simulink model "T_DARM_Functional_Architecture"  (R2021a)
settings: Solver=VariableStepAuto  StartTime=0.0  StopTime=10.0  RelTol=1e-3
settings Model: Creator=Daniel Adejumo  LastModifiedBy=Daniel Adejumo

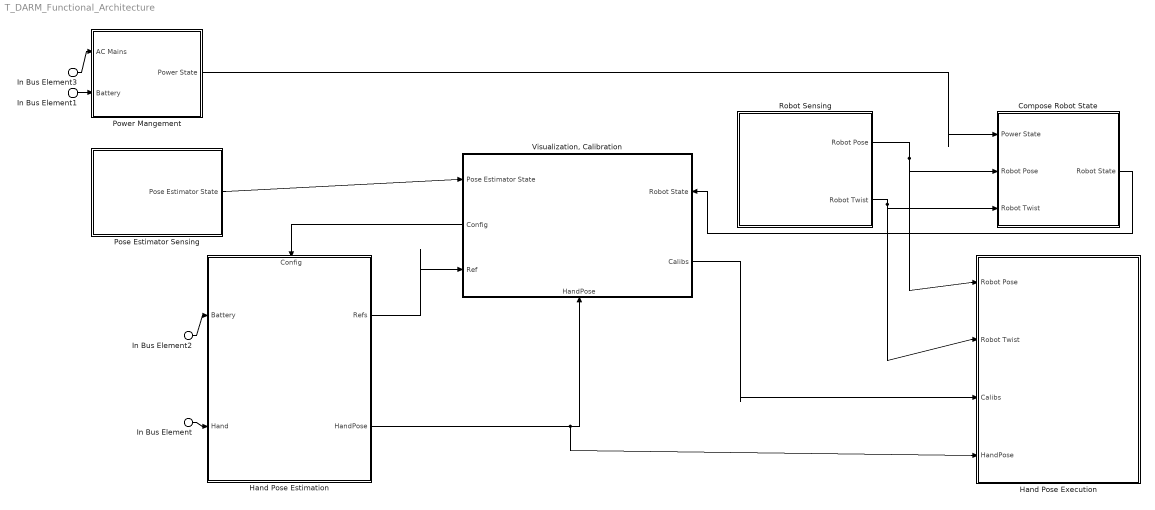
== system T_DARM_Functional_Architecture ==
  In Bus Element3 : Inport  PortName=AC Mains
  In Bus Element2 : Inport  Port=2  PortName=Battery
  In Bus Element1 : Inport  Port=2  PortName=Battery
  In Bus Element : Inport  Port=3  PortName=Hand
  Compose Robot State : Subsystem
      settings: PortSchema="{\"entries\":[{\"content\":{\"headerSize\":26,\"margin\":15,\"minimumSpacing\":25,\"sides\":[{\"content\":{\"connectorIds\":[\"In1\",\"In2\",\"In3\"]},\"type\":\"ConnectorPlacement.EquallySpacedRectSide\",\"uuid\":\"05d6e9f9-85ca-4a6e-a9b5-67e652ad81e0\"},{\"content\":{\"connectorIds\":[\"Out1\"],\"side\":\"RIGHT\"},\"type\":\"ConnectorPlacement.EquallySpacedRectSide\",\"uuid\":\"e4d931d8-63a7-4c55-9fa4-e3388543b788\"},{\"content\":{\"connectorIds\":[],\"side\":\"TOP\"},\"type\":\"ConnectorPlacement.EquallySpacedRectSide\",\"uuid\":\"0b7a612c-5d49-405f-8f52-91f0f155fa8d\"}]},\"type\":\"ConnectorPlacement.EquallySpacedConnector\",\"uuid\":\"d040a7c1-518a-4586-9505-55d0b93cd332\"}],\"packageUris\":[\"http://schema.mathworks.com/mf0/Connector/R2020b\"],\"version\":\"1.0\"}"
  Hand Pose Estimation : Subsystem
      settings: PortSchema="{\"entries\":[{\"content\":{\"headerSize\":26,\"margin\":15,\"minimumSpacing\":25,\"sides\":[{\"content\":{\"connectorIds\":[\"In2\",\"In3\"]},\"type\":\"ConnectorPlacement.EquallySpacedRectSide\",\"uuid\":\"05d6e9f9-85ca-4a6e-a9b5-67e652ad81e0\"},{\"content\":{\"connectorIds\":[\"Out1\",\"Out2\"],\"side\":\"RIGHT\"},\"type\":\"ConnectorPlacement.EquallySpacedRectSide\",\"uuid\":\"e4d931d8-63a7-4c55-9fa4-e3388543b788\"},{\"content\":{\"connectorIds\":[\"In1\"],\"side\":\"TOP\"},\"type\":\"ConnectorPlacement.EquallySpacedRectSide\",\"uuid\":\"0b7a612c-5d49-405f-8f52-91f0f155fa8d\"}]},\"type\":\"ConnectorPlacement.EquallySpacedConnector\",\"uuid\":\"d040a7c1-518a-4586-9505-55d0b93cd332\"}],\"packageUris\":[\"http://schema.mathworks.com/mf0/Connector/R2020b\"],\"version\":\"1.0\"}"
  Hand Pose Execution : Subsystem
      settings: PortSchema="{\"entries\":[{\"content\":{\"headerSize\":26,\"margin\":15,\"minimumSpacing\":25,\"sides\":[{\"content\":{\"connectorIds\":[\"In1\",\"In2\",\"In3\",\"In4\"]},\"type\":\"ConnectorPlacement.EquallySpacedRectSide\",\"uuid\":\"05d6e9f9-85ca-4a6e-a9b5-67e652ad81e0\"},{\"content\":{\"connectorIds\":[],\"side\":\"RIGHT\"},\"type\":\"ConnectorPlacement.EquallySpacedRectSide\",\"uuid\":\"e4d931d8-63a7-4c55-9fa4-e3388543b788\"},{\"content\":{\"connectorIds\":[],\"side\":\"TOP\"},\"type\":\"ConnectorPlacement.EquallySpacedRectSide\",\"uuid\":\"0b7a612c-5d49-405f-8f52-91f0f155fa8d\"}]},\"type\":\"ConnectorPlacement.EquallySpacedConnector\",\"uuid\":\"d040a7c1-518a-4586-9505-55d0b93cd332\"}],\"packageUris\":[\"http://schema.mathworks.com/mf0/Connector/R2020b\"],\"version\":\"1.0\"}"
  Pose Estimator Sensing : Subsystem
      settings: PortSchema="{\"entries\":[{\"content\":{\"headerSize\":26,\"margin\":15,\"minimumSpacing\":25,\"sides\":[{\"content\":{\"connectorIds\":[]},\"type\":\"ConnectorPlacement.EquallySpacedRectSide\",\"uuid\":\"05d6e9f9-85ca-4a6e-a9b5-67e652ad81e0\"},{\"content\":{\"connectorIds\":[\"Out1\"],\"side\":\"RIGHT\"},\"type\":\"ConnectorPlacement.EquallySpacedRectSide\",\"uuid\":\"e4d931d8-63a7-4c55-9fa4-e3388543b788\"},{\"content\":{\"connectorIds\":[],\"side\":\"TOP\"},\"type\":\"ConnectorPlacement.EquallySpacedRectSide\",\"uuid\":\"0b7a612c-5d49-405f-8f52-91f0f155fa8d\"}]},\"type\":\"ConnectorPlacement.EquallySpacedConnector\",\"uuid\":\"d040a7c1-518a-4586-9505-55d0b93cd332\"}],\"packageUris\":[\"http://schema.mathworks.com/mf0/Connector/R2020b\"],\"version\":\"1.0\"}"
  Power Mangement : Subsystem
      settings: PortSchema="{\"entries\":[{\"content\":{\"headerSize\":26,\"margin\":15,\"minimumSpacing\":25,\"sides\":[{\"content\":{\"connectorIds\":[\"In1\",\"In2\"]},\"type\":\"ConnectorPlacement.EquallySpacedRectSide\",\"uuid\":\"05d6e9f9-85ca-4a6e-a9b5-67e652ad81e0\"},{\"content\":{\"connectorIds\":[\"Out1\"],\"side\":\"RIGHT\"},\"type\":\"ConnectorPlacement.EquallySpacedRectSide\",\"uuid\":\"e4d931d8-63a7-4c55-9fa4-e3388543b788\"},{\"content\":{\"connectorIds\":[],\"side\":\"TOP\"},\"type\":\"ConnectorPlacement.EquallySpacedRectSide\",\"uuid\":\"0b7a612c-5d49-405f-8f52-91f0f155fa8d\"}]},\"type\":\"ConnectorPlacement.EquallySpacedConnector\",\"uuid\":\"d040a7c1-518a-4586-9505-55d0b93cd332\"}],\"packageUris\":[\"http://schema.mathworks.com/mf0/Connector/R2020b\"],\"version\":\"1.0\"}"
  Robot Sensing : Subsystem
      settings: PortSchema="{\"entries\":[{\"content\":{\"headerSize\":26,\"margin\":15,\"minimumSpacing\":25,\"sides\":[{\"content\":{\"connectorIds\":[]},\"type\":\"ConnectorPlacement.EquallySpacedRectSide\",\"uuid\":\"05d6e9f9-85ca-4a6e-a9b5-67e652ad81e0\"},{\"content\":{\"connectorIds\":[\"Out1\",\"Out2\"],\"side\":\"RIGHT\"},\"type\":\"ConnectorPlacement.EquallySpacedRectSide\",\"uuid\":\"e4d931d8-63a7-4c55-9fa4-e3388543b788\"},{\"content\":{\"connectorIds\":[],\"side\":\"TOP\"},\"type\":\"ConnectorPlacement.EquallySpacedRectSide\",\"uuid\":\"0b7a612c-5d49-405f-8f52-91f0f155fa8d\"}]},\"type\":\"ConnectorPlacement.EquallySpacedConnector\",\"uuid\":\"d040a7c1-518a-4586-9505-55d0b93cd332\"}],\"packageUris\":[\"http://schema.mathworks.com/mf0/Connector/R2020b\"],\"version\":\"1.0\"}"
  "Visualization, Calibration" : Subsystem
      settings: PortSchema="{\"entries\":[{\"content\":{\"headerSize\":26,\"margin\":15,\"minimumSpacing\":25,\"sides\":[{\"content\":{\"connectorIds\":[\"In2\",\"Out1\",\"In3\"]},\"type\":\"ConnectorPlacement.EquallySpacedRectSide\",\"uuid\":\"05d6e9f9-85ca-4a6e-a9b5-67e652ad81e0\"},{\"content\":{\"connectorIds\":[\"In1\",\"Out2\"],\"side\":\"RIGHT\"},\"type\":\"ConnectorPlacement.EquallySpacedRectSide\",\"uuid\":\"e4d931d8-63a7-4c55-9fa4-e3388543b788\"},{\"content\":{\"connectorIds\":[],\"side\":\"TOP\"},\"type\":\"ConnectorPlacement.EquallySpacedRectSide\",\"uuid\":\"0b7a612c-5d49-405f-8f52-91f0f155fa8d\"},{\"content\":{\"connectorIds\":[\"In4\"],\"side\":\"BOTTOM\"},\"type\":\"ConnectorPlacement.EquallySpacedRectSide\",\"uuid\":\"e4f71b4a-9bde-4719-ae21-9a20012d87c4\"}]},\"type\":\"ConnectorPlacement.EquallySpacedConnector\",\"uuid\":\"d040a7c1-518a-4586-9505-55d0b93cd332\"}],\"packageUris\":[\"http://schema.mathworks.com/mf0/Connector/R2020b\"],\"version\":\"1.0\"}"
  wires:
  In Bus Element/1 -> Hand Pose Estimation/3(Hand)
  Hand Pose Estimation/2(HandPose) -> "Visualization, Calibration"/4(HandPose), Hand Pose Execution/4(HandPose)
  In Bus Element2/1 -> Hand Pose Estimation/2(Battery)
  Hand Pose Estimation/1(Refs) -> "Visualization, Calibration"/3(Ref)
  "Visualization, Calibration"/2(Calibs) -> Hand Pose Execution/3(Calibs)
  "Visualization, Calibration"/1(Config) -> Hand Pose Estimation/1(Config)
  In Bus Element3/1 -> Power Mangement/1(AC Mains)
  Robot Sensing/2(Robot Twist) -> Hand Pose Execution/2(Robot Twist), Compose Robot State/3(Robot Twist)
  Robot Sensing/1(Robot Pose) -> Hand Pose Execution/1(Robot Pose), Compose Robot State/2(Robot Pose)
  Compose Robot State/1(Robot State) -> "Visualization, Calibration"/1(Robot State)
  Power Mangement/1(Power State) -> Compose Robot State/1(Power State)
  Pose Estimator Sensing/1(Pose Estimator State) -> "Visualization, Calibration"/2(Pose Estimator State)
  In Bus Element1/1 -> Power Mangement/2(Battery)

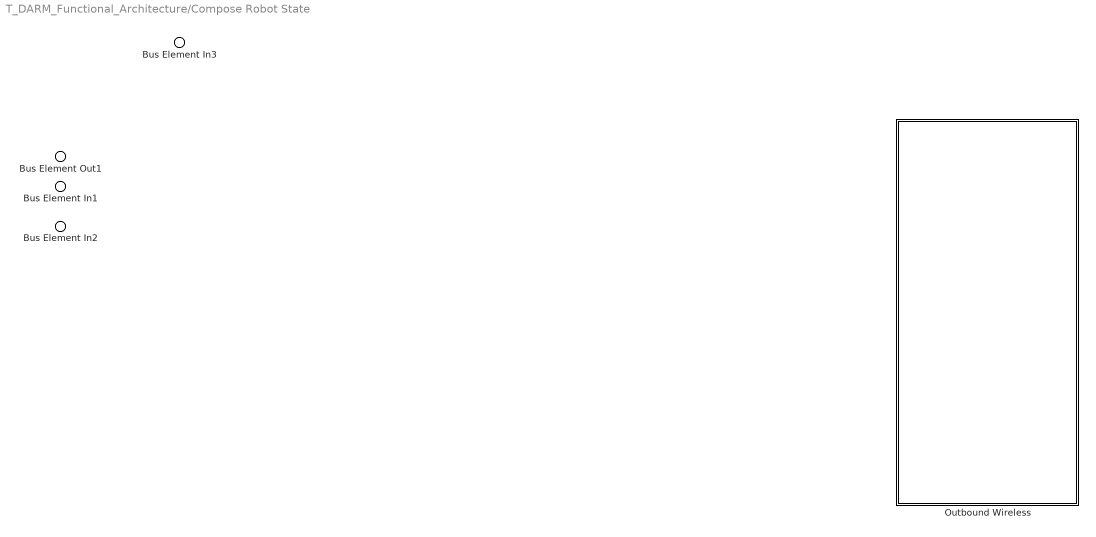
== system T_DARM_Functional_Architecture/Compose Robot State ==
  Bus Element In3 : Inport  PortName=Power State
  Bus Element In1 : Inport  Port=2  PortName=Robot Pose
  Bus Element In2 : Inport  Port=3  PortName=Robot Twist
  Outbound Wireless : Subsystem
      settings: PortSchema="{\"entries\":[{\"content\":{\"headerSize\":26,\"margin\":15,\"minimumSpacing\":25,\"sides\":[{\"content\":{\"connectorIds\":[]},\"type\":\"ConnectorPlacement.EquallySpacedRectSide\",\"uuid\":\"05d6e9f9-85ca-4a6e-a9b5-67e652ad81e0\"},{\"content\":{\"connectorIds\":[],\"side\":\"RIGHT\"},\"type\":\"ConnectorPlacement.EquallySpacedRectSide\",\"uuid\":\"e4d931d8-63a7-4c55-9fa4-e3388543b788\"},{\"content\":{\"connectorIds\":[],\"side\":\"TOP\"},\"type\":\"ConnectorPlacement.EquallySpacedRectSide\",\"uuid\":\"0b7a612c-5d49-405f-8f52-91f0f155fa8d\"}]},\"type\":\"ConnectorPlacement.EquallySpacedConnector\",\"uuid\":\"d040a7c1-518a-4586-9505-55d0b93cd332\"}],\"packageUris\":[\"http://schema.mathworks.com/mf0/Connector/R2020b\"],\"version\":\"1.0\"}"
  Bus Element Out1 : Outport  PortName=Robot State

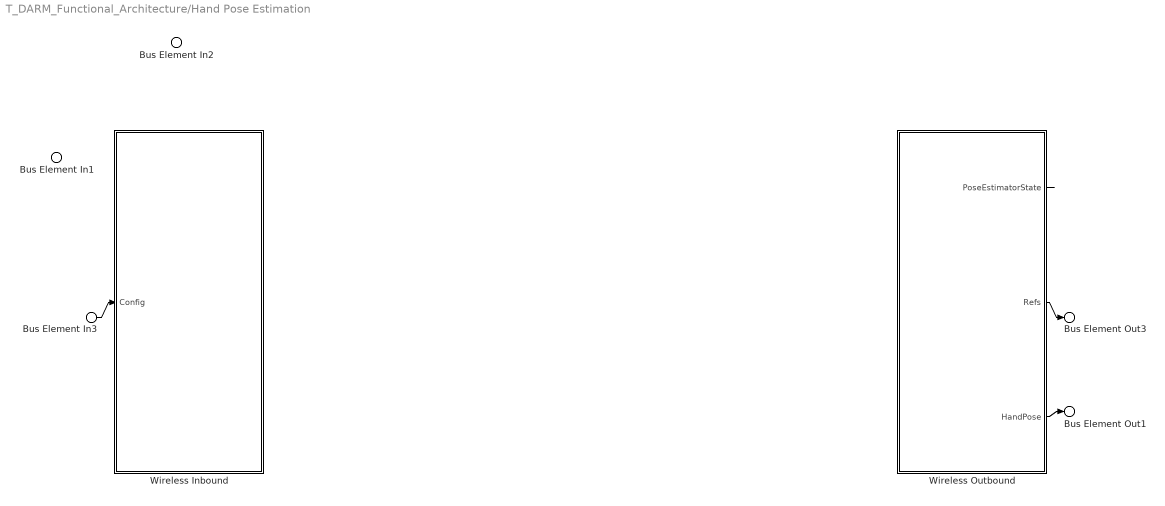
== system T_DARM_Functional_Architecture/Hand Pose Estimation ==
  Bus Element In3 : Inport  PortName=Config
  Bus Element In2 : Inport  Port=2  PortName=Battery
  Bus Element In1 : Inport  Port=3  PortName=Hand
  Wireless Inbound : Subsystem
      settings: PortSchema="{\"entries\":[{\"content\":{\"headerSize\":26,\"margin\":15,\"minimumSpacing\":25,\"sides\":[{\"content\":{\"connectorIds\":[\"In1\"]},\"type\":\"ConnectorPlacement.EquallySpacedRectSide\",\"uuid\":\"05d6e9f9-85ca-4a6e-a9b5-67e652ad81e0\"},{\"content\":{\"connectorIds\":[],\"side\":\"RIGHT\"},\"type\":\"ConnectorPlacement.EquallySpacedRectSide\",\"uuid\":\"e4d931d8-63a7-4c55-9fa4-e3388543b788\"},{\"content\":{\"connectorIds\":[],\"side\":\"TOP\"},\"type\":\"ConnectorPlacement.EquallySpacedRectSide\",\"uuid\":\"0b7a612c-5d49-405f-8f52-91f0f155fa8d\"}]},\"type\":\"ConnectorPlacement.EquallySpacedConnector\",\"uuid\":\"d040a7c1-518a-4586-9505-55d0b93cd332\"}],\"packageUris\":[\"http://schema.mathworks.com/mf0/Connector/R2020b\"],\"version\":\"1.0\"}"
  Wireless Outbound : Subsystem
      settings: PortSchema="{\"entries\":[{\"content\":{\"headerSize\":26,\"margin\":15,\"minimumSpacing\":25,\"sides\":[{\"content\":{\"connectorIds\":[]},\"type\":\"ConnectorPlacement.EquallySpacedRectSide\",\"uuid\":\"05d6e9f9-85ca-4a6e-a9b5-67e652ad81e0\"},{\"content\":{\"connectorIds\":[\"Out1\",\"Out2\",\"Out3\"],\"side\":\"RIGHT\"},\"type\":\"ConnectorPlacement.EquallySpacedRectSide\",\"uuid\":\"e4d931d8-63a7-4c55-9fa4-e3388543b788\"},{\"content\":{\"connectorIds\":[],\"side\":\"TOP\"},\"type\":\"ConnectorPlacement.EquallySpacedRectSide\",\"uuid\":\"0b7a612c-5d49-405f-8f52-91f0f155fa8d\"}]},\"type\":\"ConnectorPlacement.EquallySpacedConnector\",\"uuid\":\"d040a7c1-518a-4586-9505-55d0b93cd332\"}],\"packageUris\":[\"http://schema.mathworks.com/mf0/Connector/R2020b\"],\"version\":\"1.0\"}"
  Bus Element Out3 : Outport  PortName=Refs
  Bus Element Out1 : Outport  Port=2  PortName=HandPose
  wires:
  Wireless Outbound/1(PoseEstimatorState) -> ?
  Wireless Outbound/2(Refs) -> Bus Element Out3/1
  Wireless Outbound/3(HandPose) -> Bus Element Out1/1
  Bus Element In3/1 -> Wireless Inbound/1(Config)

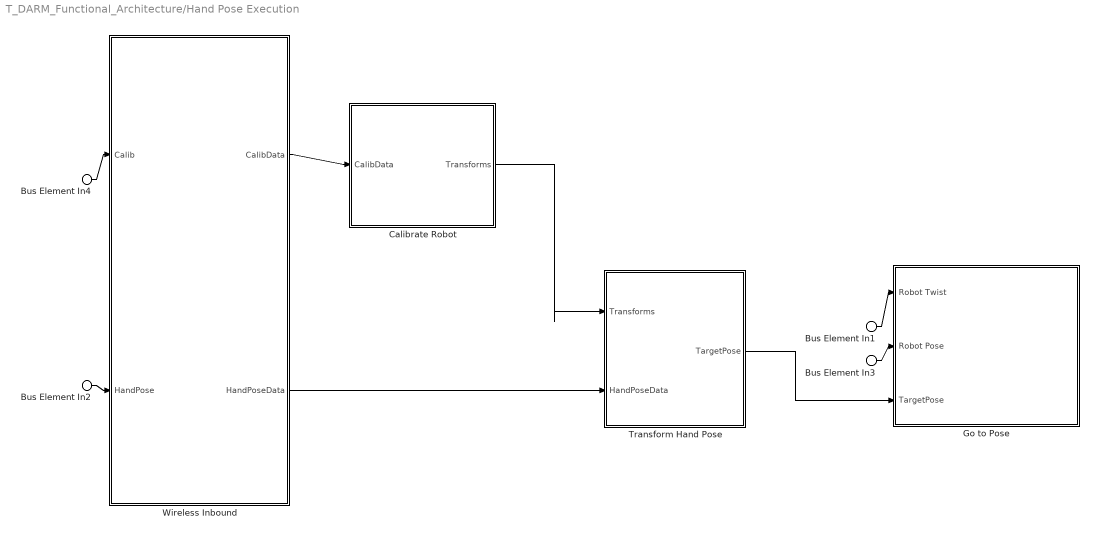
== system T_DARM_Functional_Architecture/Hand Pose Execution ==
  Bus Element In3 : Inport  PortName=Robot Pose
  Bus Element In1 : Inport  Port=2  PortName=Robot Twist
  Bus Element In4 : Inport  Port=3  PortName=Calibs
  Bus Element In2 : Inport  Port=4  PortName=HandPose
  Calibrate Robot : Subsystem
      settings: PortSchema="{\"entries\":[{\"content\":{\"headerSize\":26,\"margin\":15,\"minimumSpacing\":25,\"sides\":[{\"content\":{\"connectorIds\":[\"In1\"]},\"type\":\"ConnectorPlacement.EquallySpacedRectSide\",\"uuid\":\"05d6e9f9-85ca-4a6e-a9b5-67e652ad81e0\"},{\"content\":{\"connectorIds\":[\"Out1\"],\"side\":\"RIGHT\"},\"type\":\"ConnectorPlacement.EquallySpacedRectSide\",\"uuid\":\"e4d931d8-63a7-4c55-9fa4-e3388543b788\"},{\"content\":{\"connectorIds\":[],\"side\":\"TOP\"},\"type\":\"ConnectorPlacement.EquallySpacedRectSide\",\"uuid\":\"0b7a612c-5d49-405f-8f52-91f0f155fa8d\"}]},\"type\":\"ConnectorPlacement.EquallySpacedConnector\",\"uuid\":\"d040a7c1-518a-4586-9505-55d0b93cd332\"}],\"packageUris\":[\"http://schema.mathworks.com/mf0/Connector/R2020b\"],\"version\":\"1.0\"}"
  Go to Pose : Subsystem
      settings: PortSchema="{\"entries\":[{\"content\":{\"headerSize\":26,\"margin\":15,\"minimumSpacing\":25,\"sides\":[{\"content\":{\"connectorIds\":[\"In2\",\"In3\",\"In1\"]},\"type\":\"ConnectorPlacement.EquallySpacedRectSide\",\"uuid\":\"05d6e9f9-85ca-4a6e-a9b5-67e652ad81e0\"},{\"content\":{\"connectorIds\":[],\"side\":\"RIGHT\"},\"type\":\"ConnectorPlacement.EquallySpacedRectSide\",\"uuid\":\"e4d931d8-63a7-4c55-9fa4-e3388543b788\"},{\"content\":{\"connectorIds\":[],\"side\":\"TOP\"},\"type\":\"ConnectorPlacement.EquallySpacedRectSide\",\"uuid\":\"0b7a612c-5d49-405f-8f52-91f0f155fa8d\"}]},\"type\":\"ConnectorPlacement.EquallySpacedConnector\",\"uuid\":\"d040a7c1-518a-4586-9505-55d0b93cd332\"}],\"packageUris\":[\"http://schema.mathworks.com/mf0/Connector/R2020b\"],\"version\":\"1.0\"}"
  Transform Hand Pose : Subsystem
      settings: PortSchema="{\"entries\":[{\"content\":{\"headerSize\":26,\"margin\":15,\"minimumSpacing\":25,\"sides\":[{\"content\":{\"connectorIds\":[\"In1\",\"In2\"]},\"type\":\"ConnectorPlacement.EquallySpacedRectSide\",\"uuid\":\"05d6e9f9-85ca-4a6e-a9b5-67e652ad81e0\"},{\"content\":{\"connectorIds\":[\"Out1\"],\"side\":\"RIGHT\"},\"type\":\"ConnectorPlacement.EquallySpacedRectSide\",\"uuid\":\"e4d931d8-63a7-4c55-9fa4-e3388543b788\"},{\"content\":{\"connectorIds\":[],\"side\":\"TOP\"},\"type\":\"ConnectorPlacement.EquallySpacedRectSide\",\"uuid\":\"0b7a612c-5d49-405f-8f52-91f0f155fa8d\"}]},\"type\":\"ConnectorPlacement.EquallySpacedConnector\",\"uuid\":\"d040a7c1-518a-4586-9505-55d0b93cd332\"}],\"packageUris\":[\"http://schema.mathworks.com/mf0/Connector/R2020b\"],\"version\":\"1.0\"}"
  Wireless Inbound : Subsystem
      settings: PortSchema="{\"entries\":[{\"content\":{\"headerSize\":26,\"margin\":15,\"minimumSpacing\":25,\"sides\":[{\"content\":{\"connectorIds\":[\"In1\",\"In2\"]},\"type\":\"ConnectorPlacement.EquallySpacedRectSide\",\"uuid\":\"05d6e9f9-85ca-4a6e-a9b5-67e652ad81e0\"},{\"content\":{\"connectorIds\":[\"Out1\",\"Out2\"],\"side\":\"RIGHT\"},\"type\":\"ConnectorPlacement.EquallySpacedRectSide\",\"uuid\":\"e4d931d8-63a7-4c55-9fa4-e3388543b788\"},{\"content\":{\"connectorIds\":[],\"side\":\"TOP\"},\"type\":\"ConnectorPlacement.EquallySpacedRectSide\",\"uuid\":\"0b7a612c-5d49-405f-8f52-91f0f155fa8d\"}]},\"type\":\"ConnectorPlacement.EquallySpacedConnector\",\"uuid\":\"d040a7c1-518a-4586-9505-55d0b93cd332\"}],\"packageUris\":[\"http://schema.mathworks.com/mf0/Connector/R2020b\"],\"version\":\"1.0\"}"
  wires:
  Calibrate Robot/1(Transforms) -> Transform Hand Pose/1(Transforms)
  Transform Hand Pose/1(TargetPose) -> Go to Pose/1(TargetPose)
  Bus Element In4/1 -> Wireless Inbound/1(Calib)
  Bus Element In2/1 -> Wireless Inbound/2(HandPose)
  Wireless Inbound/1(CalibData) -> Calibrate Robot/1(CalibData)
  Wireless Inbound/2(HandPoseData) -> Transform Hand Pose/2(HandPoseData)
  Bus Element In1/1 -> Go to Pose/2(Robot Twist)
  Bus Element In3/1 -> Go to Pose/3(Robot Pose)

== system T_DARM_Functional_Architecture/Pose Estimator Sensing ==
  Bus Element Out1 : Outport  PortName=Pose Estimator State

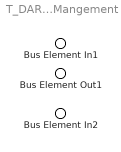
== system T_DARM_Functional_Architecture/Power Mangement ==
  Bus Element In1 : Inport  PortName=AC Mains
  Bus Element In2 : Inport  Port=2  PortName=Battery
  Bus Element Out1 : Outport  PortName=Power State

== system T_DARM_Functional_Architecture/Robot Sensing ==
  Bus Element Out1 : Outport  PortName=Robot Pose
  Bus Element Out2 : Outport  Port=2  PortName=Robot Twist

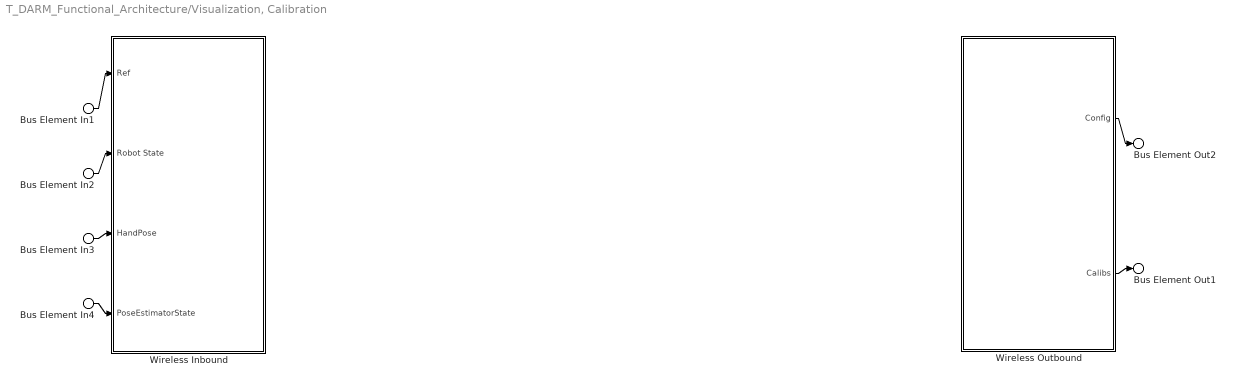
== system T_DARM_Functional_Architecture/Visualization, Calibration ==
  Bus Element In2 : Inport  PortName=Robot State
  Bus Element In4 : Inport  Port=2  PortName=Pose Estimator State
  Bus Element In1 : Inport  Port=3  PortName=Ref
  Bus Element In3 : Inport  Port=4  PortName=HandPose
  Wireless Inbound : Subsystem
      settings: PortSchema="{\"entries\":[{\"content\":{\"headerSize\":26,\"margin\":15,\"minimumSpacing\":25,\"sides\":[{\"content\":{\"connectorIds\":[\"In4\",\"In2\",\"In3\",\"In1\"]},\"type\":\"ConnectorPlacement.EquallySpacedRectSide\",\"uuid\":\"05d6e9f9-85ca-4a6e-a9b5-67e652ad81e0\"},{\"content\":{\"connectorIds\":[],\"side\":\"RIGHT\"},\"type\":\"ConnectorPlacement.EquallySpacedRectSide\",\"uuid\":\"e4d931d8-63a7-4c55-9fa4-e3388543b788\"},{\"content\":{\"connectorIds\":[],\"side\":\"TOP\"},\"type\":\"ConnectorPlacement.EquallySpacedRectSide\",\"uuid\":\"0b7a612c-5d49-405f-8f52-91f0f155fa8d\"}]},\"type\":\"ConnectorPlacement.EquallySpacedConnector\",\"uuid\":\"d040a7c1-518a-4586-9505-55d0b93cd332\"}],\"packageUris\":[\"http://schema.mathworks.com/mf0/Connector/R2020b\"],\"version\":\"1.0\"}"
  Wireless Outbound : Subsystem
      settings: PortSchema="{\"entries\":[{\"content\":{\"headerSize\":26,\"margin\":15,\"minimumSpacing\":25,\"sides\":[{\"content\":{\"connectorIds\":[]},\"type\":\"ConnectorPlacement.EquallySpacedRectSide\",\"uuid\":\"05d6e9f9-85ca-4a6e-a9b5-67e652ad81e0\"},{\"content\":{\"connectorIds\":[\"Out1\",\"Out2\"],\"side\":\"RIGHT\"},\"type\":\"ConnectorPlacement.EquallySpacedRectSide\",\"uuid\":\"e4d931d8-63a7-4c55-9fa4-e3388543b788\"},{\"content\":{\"connectorIds\":[],\"side\":\"TOP\"},\"type\":\"ConnectorPlacement.EquallySpacedRectSide\",\"uuid\":\"0b7a612c-5d49-405f-8f52-91f0f155fa8d\"}]},\"type\":\"ConnectorPlacement.EquallySpacedConnector\",\"uuid\":\"d040a7c1-518a-4586-9505-55d0b93cd332\"}],\"packageUris\":[\"http://schema.mathworks.com/mf0/Connector/R2020b\"],\"version\":\"1.0\"}"
  Bus Element Out2 : Outport  PortName=Config
  Bus Element Out1 : Outport  Port=2  PortName=Calibs
  wires:
  Bus Element In4/1 -> Wireless Inbound/1(PoseEstimatorState)
  Bus Element In1/1 -> Wireless Inbound/4(Ref)
  Bus Element In3/1 -> Wireless Inbound/3(HandPose)
  Wireless Outbound/1(Config) -> Bus Element Out2/1
  Wireless Outbound/2(Calibs) -> Bus Element Out1/1
  Bus Element In2/1 -> Wireless Inbound/2(Robot State)

== system T_DARM_Functional_Architecture/Compose Robot State/Outbound Wireless ==

== system T_DARM_Functional_Architecture/Hand Pose Estimation/Wireless Inbound ==
  Bus Element In1 : Inport  PortName=Config

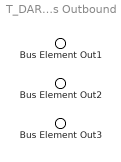
== system T_DARM_Functional_Architecture/Hand Pose Estimation/Wireless Outbound ==
  Bus Element Out1 : Outport  PortName=PoseEstimatorState
  Bus Element Out2 : Outport  Port=2  PortName=Refs
  Bus Element Out3 : Outport  Port=3  PortName=HandPose

== system T_DARM_Functional_Architecture/Hand Pose Execution/Calibrate Robot ==
  Bus Element In1 : Inport  PortName=CalibData
  Bus Element Out1 : Outport  PortName=Transforms

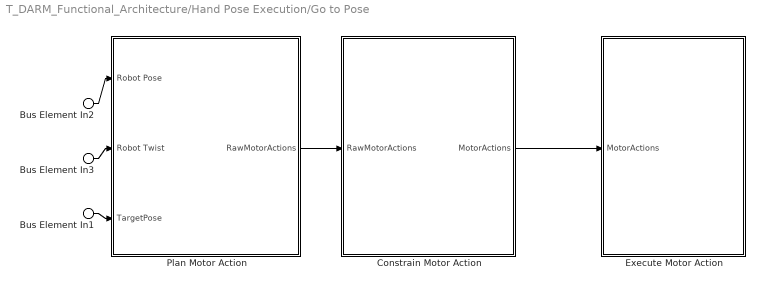
== system T_DARM_Functional_Architecture/Hand Pose Execution/Go to Pose ==
  Bus Element In1 : Inport  PortName=TargetPose
  Bus Element In3 : Inport  Port=2  PortName=Robot Twist
  Bus Element In2 : Inport  Port=3  PortName=Robot Pose
  Constrain Motor Action : Subsystem
      settings: PortSchema="{\"entries\":[{\"content\":{\"headerSize\":26,\"margin\":15,\"minimumSpacing\":25,\"sides\":[{\"content\":{\"connectorIds\":[\"In1\"]},\"type\":\"ConnectorPlacement.EquallySpacedRectSide\",\"uuid\":\"05d6e9f9-85ca-4a6e-a9b5-67e652ad81e0\"},{\"content\":{\"connectorIds\":[\"Out1\"],\"side\":\"RIGHT\"},\"type\":\"ConnectorPlacement.EquallySpacedRectSide\",\"uuid\":\"e4d931d8-63a7-4c55-9fa4-e3388543b788\"},{\"content\":{\"connectorIds\":[],\"side\":\"TOP\"},\"type\":\"ConnectorPlacement.EquallySpacedRectSide\",\"uuid\":\"0b7a612c-5d49-405f-8f52-91f0f155fa8d\"}]},\"type\":\"ConnectorPlacement.EquallySpacedConnector\",\"uuid\":\"d040a7c1-518a-4586-9505-55d0b93cd332\"}],\"packageUris\":[\"http://schema.mathworks.com/mf0/Connector/R2020b\"],\"version\":\"1.0\"}"
  Execute Motor Action : Subsystem
      settings: PortSchema="{\"entries\":[{\"content\":{\"headerSize\":26,\"margin\":15,\"minimumSpacing\":25,\"sides\":[{\"content\":{\"connectorIds\":[\"In1\"]},\"type\":\"ConnectorPlacement.EquallySpacedRectSide\",\"uuid\":\"05d6e9f9-85ca-4a6e-a9b5-67e652ad81e0\"},{\"content\":{\"connectorIds\":[],\"side\":\"RIGHT\"},\"type\":\"ConnectorPlacement.EquallySpacedRectSide\",\"uuid\":\"e4d931d8-63a7-4c55-9fa4-e3388543b788\"},{\"content\":{\"connectorIds\":[],\"side\":\"TOP\"},\"type\":\"ConnectorPlacement.EquallySpacedRectSide\",\"uuid\":\"0b7a612c-5d49-405f-8f52-91f0f155fa8d\"}]},\"type\":\"ConnectorPlacement.EquallySpacedConnector\",\"uuid\":\"d040a7c1-518a-4586-9505-55d0b93cd332\"}],\"packageUris\":[\"http://schema.mathworks.com/mf0/Connector/R2020b\"],\"version\":\"1.0\"}"
  Plan Motor Action : Subsystem
      settings: PortSchema="{\"entries\":[{\"content\":{\"headerSize\":26,\"margin\":15,\"minimumSpacing\":25,\"sides\":[{\"content\":{\"connectorIds\":[\"In1\",\"In2\",\"In3\"]},\"type\":\"ConnectorPlacement.EquallySpacedRectSide\",\"uuid\":\"05d6e9f9-85ca-4a6e-a9b5-67e652ad81e0\"},{\"content\":{\"connectorIds\":[\"Out1\"],\"side\":\"RIGHT\"},\"type\":\"ConnectorPlacement.EquallySpacedRectSide\",\"uuid\":\"e4d931d8-63a7-4c55-9fa4-e3388543b788\"},{\"content\":{\"connectorIds\":[],\"side\":\"TOP\"},\"type\":\"ConnectorPlacement.EquallySpacedRectSide\",\"uuid\":\"0b7a612c-5d49-405f-8f52-91f0f155fa8d\"}]},\"type\":\"ConnectorPlacement.EquallySpacedConnector\",\"uuid\":\"d040a7c1-518a-4586-9505-55d0b93cd332\"}],\"packageUris\":[\"http://schema.mathworks.com/mf0/Connector/R2020b\"],\"version\":\"1.0\"}"
  wires:
  Plan Motor Action/1(RawMotorActions) -> Constrain Motor Action/1(RawMotorActions)
  Constrain Motor Action/1(MotorActions) -> Execute Motor Action/1(MotorActions)
  Bus Element In1/1 -> Plan Motor Action/3(TargetPose)
  Bus Element In2/1 -> Plan Motor Action/1(Robot Pose)
  Bus Element In3/1 -> Plan Motor Action/2(Robot Twist)

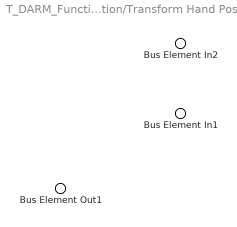
== system T_DARM_Functional_Architecture/Hand Pose Execution/Transform Hand Pose ==
  Bus Element In2 : Inport  PortName=Transforms
  Bus Element In1 : Inport  Port=2  PortName=HandPoseData
  Bus Element Out1 : Outport  PortName=TargetPose

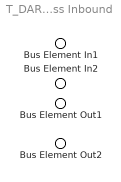
== system T_DARM_Functional_Architecture/Hand Pose Execution/Wireless Inbound ==
  Bus Element In1 : Inport  PortName=Calib
  Bus Element In2 : Inport  Port=2  PortName=HandPose
  Bus Element Out1 : Outport  PortName=CalibData
  Bus Element Out2 : Outport  Port=2  PortName=HandPoseData

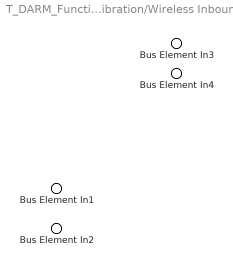
== system T_DARM_Functional_Architecture/Visualization, Calibration/Wireless Inbound ==
  Bus Element In1 : Inport  PortName=PoseEstimatorState
  Bus Element In4 : Inport  Port=2  PortName=Robot State
  Bus Element In3 : Inport  Port=3  PortName=HandPose
  Bus Element In2 : Inport  Port=4  PortName=Ref

== system T_DARM_Functional_Architecture/Visualization, Calibration/Wireless Outbound ==
  Bus Element Out1 : Outport  PortName=Config
  Bus Element Out2 : Outport  Port=2  PortName=Calibs

== system T_DARM_Functional_Architecture/Hand Pose Execution/Go to Pose/Constrain Motor Action ==
  Bus Element In1 : Inport  PortName=RawMotorActions
  Bus Element Out1 : Outport  PortName=MotorActions

== system T_DARM_Functional_Architecture/Hand Pose Execution/Go to Pose/Execute Motor Action ==
  Bus Element In1 : Inport  PortName=MotorActions

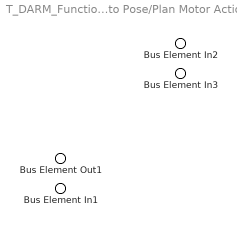
== system T_DARM_Functional_Architecture/Hand Pose Execution/Go to Pose/Plan Motor Action ==
  Bus Element In3 : Inport  PortName=Robot Pose
  Bus Element In2 : Inport  Port=2  PortName=Robot Twist
  Bus Element In1 : Inport  Port=3  PortName=TargetPose
  Bus Element Out1 : Outport  PortName=RawMotorActions
